simulink subsystem "aeroForces"  (R2023b)
settings: Solver=VariableStepAuto  StartTime=0.0  StopTime=10.0  RelTol=1e-3
undefined symbols (not defined in the file): b, c, rho, S_wing
libraries: sharedtransform x1
settings Model: Creator=Victor  LastModifiedBy=Victor

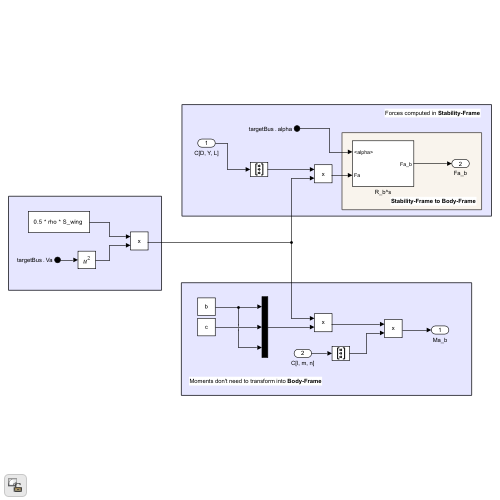
[thumbnail: Simulink's stored preview of the top-level diagram]
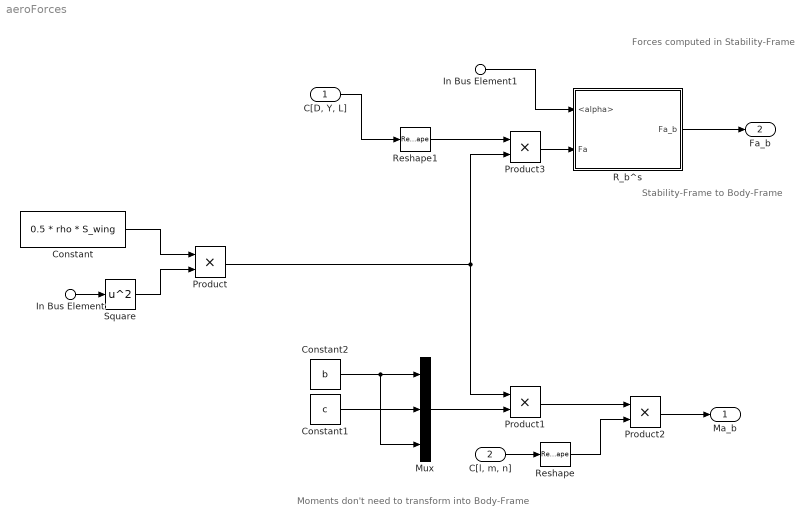
== system aeroForces ==
  note: Moments don't need to transform into Body-Frame
  note: Forces computed in Stability-Frame
  note: Stability-Frame to Body-Frame
  "C[D, Y, L]" : Inport
  "C[l, m, n]" : Inport  Port=2
  In Bus Element : Inport  Port=3  PortName=targetBus  Element=Va
  In Bus Element1 : Inport  Port=3  PortName=targetBus  Element=alpha
  Constant : Constant  Value=0.5 * rho * S_wing
  Constant1 : Constant  Value=c
  Constant2 : Constant  Value=b
  Mux : Mux  Inputs=3
  Product{,1..3} (4 alike) : Product
  R_b^s : Subsystem
  Reshape : Reshape  OutputDimensionality=Column vector (2-D)
  Reshape1 : Reshape  OutputDimensionality=Column vector (2-D)
  Square : Math  Operator=square
  Ma_b : Outport
  Fa_b : Outport  Port=2
  wires:
  R_b^s/1(Fa_b) -> Fa_b/1
  In Bus Element/1 -> Square/1
  Square/1 -> Product/2
  Constant/1 -> Product/1
  Constant1/1 -> Mux/2
  Constant2/1 -> Mux/1, Mux/3
  Mux/1 -> Product1/2
  "C[l, m, n]"/1 -> Reshape/1
  Product1/1 -> Product2/1
  Product2/1 -> Ma_b/1
  Product3/1 -> R_b^s/2(Fa)
  "C[D, Y, L]"/1 -> Reshape1/1
  Product/1 -> Product1/1, Product3/2
  In Bus Element1/1 -> R_b^s/1(<alpha>)
  Reshape/1 -> Product2/2
  Reshape1/1 -> Product3/1

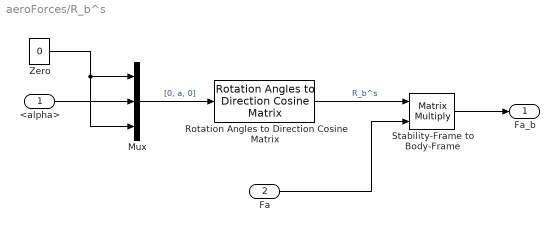
== system aeroForces/R_b^s ==
  <alpha> : Inport
  Fa : Inport  Port=2
  Mux : Mux  Inputs=3
  Rotation Angles to Direction Cosine Matrix : sharedtransform/Rotation Angles to Direction Cosine Matrix  rotationOrder=ZYX  aMode=aMode
  Stability-Frame to Body-Frame : Product  Multiplication=Matrix(*)
  Zero : Constant  Value=0  OutDataTypeStr=Inherit: Inherit via back propagation
  Fa_b : Outport
  wires:
  <alpha>/1 -> Mux/2
  Rotation Angles to Direction Cosine Matrix/1 -> Stability-Frame to Body-Frame/1  "R_b^s"
  Zero/1 -> Mux/1, Mux/3
  Mux/1 -> Rotation Angles to Direction Cosine Matrix/1  "[0, a, 0]"
  Fa/1 -> Stability-Frame to Body-Frame/2
  Stability-Frame to Body-Frame/1 -> Fa_b/1
